simulink model "seguimiento_constante_nominal_modelo_lineal_controlable"  (R2021a)
settings: Solver=VariableStepAuto  StartTime=0.0  StopTime=15  RelTol=1e-3
settings Model: Creator=jmata  LastModifiedBy=jmata

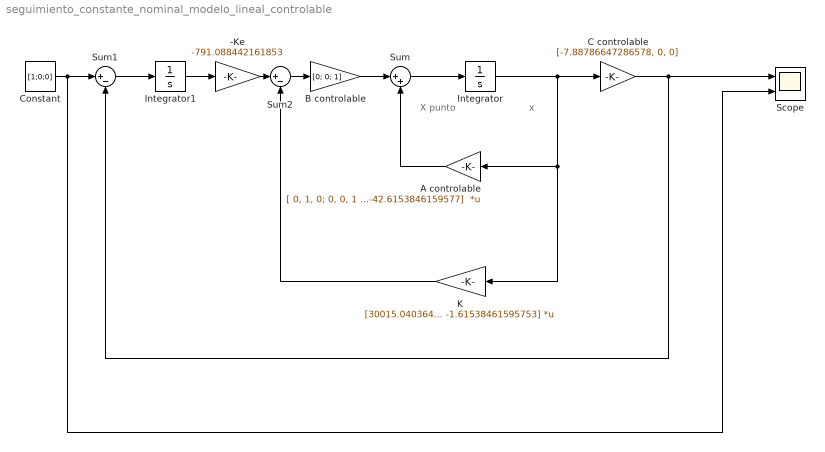
== system seguimiento_constante_nominal_modelo_lineal_controlable ==
  note: x
  note: X punto
  -Ke : Gain  Gain=-791.088442161853
  A controlable : Gain  Gain=|  Multiplication=Matrix(K*u)
      | [ 0, 1, 0; 0, 0, 1
      |  ;26809.0403648094, 629.09300494194, -42.6153846159577]
  B controlable : Gain  Gain=[0; 0; 1]
  C controlable : Gain  Gain=[-7.88786647286578, 0, 0]
  Constant : Constant  Value=[1;0;0]
  Integrator : Integrator
  Integrator1 : Integrator
  K : Gain  Gain=[30015.0403648094, 1205.0930049419, -1.61538461595753]  Multiplication=Matrix(K*u)
  Scope : Scope  NumInputPorts=2
  Sum : Sum  Inputs=|++
  Sum1 : Sum  Inputs=|+-
  Sum2 : Sum  Inputs=|+-
  wires:
  A controlable/1 -> Sum/2
  B controlable/1 -> Sum/1
  Sum/1 -> Integrator/1
  Integrator/1 -> K/1, A controlable/1, C controlable/1
  C controlable/1 -> Sum1/2, Scope/1
  Sum1/1 -> Integrator1/1
  Integrator1/1 -> -Ke/1
  -Ke/1 -> Sum2/1
  Sum2/1 -> B controlable/1
  K/1 -> Sum2/2
  Constant/1 -> Scope/2, Sum1/1
